simulink model "TorqueVectoring_6_1"  (R2023a)
settings: Solver=FixedStepAuto  StartTime=0.0  StopTime=8  FixedStep=.001  RelTol=1e-3
model workspace (MAT data in the model file):
  slipTarget : Simulink.Parameter (value not decoded)
values from neighbouring files (symbols this model uses):
  Kd_slip = 0    [Main_TorqueVectoring_5_1.m]
  Kd_yaw = 0    [Main_TorqueVectoring_5_1.m]
  Ki_slip = 50    [Main_TorqueVectoring_5_1.m]
  Ki_yaw = 10    [Main_TorqueVectoring_5_1.m]
  Kp_slip = 250    [Main_TorqueVectoring_5_1.m]
  Kp_yaw = 100    [Main_TorqueVectoring_5_1.m]
  slip_windupLower = -inf    [Main_TorqueVectoring_5_1.m]
  slip_windupUpper = inf    [Main_TorqueVectoring_5_1.m]
  slipTarget = .2    (= 0.2)    [Main_TorqueVectoring_5_1.m]
  steering = table2array(yawrateSteering)    [Main_TorqueVectoring_5_1.m]
  yaw_prev_error = 0    [Main_TorqueVectoring_5_1.m]
  yawRate = table2array(yawrateTable)    [Main_TorqueVectoring_5_1.m]
  yawrateVelocity = [0, 5, 10, 15, 20, 25, 30, 35]    [Main_TorqueVectoring_5_1.m]
undefined symbols (not defined in the file or in its folder): sigbuilder_block, VehicleVelocity
libraries: slpidlib x6
(part 2 of 4)

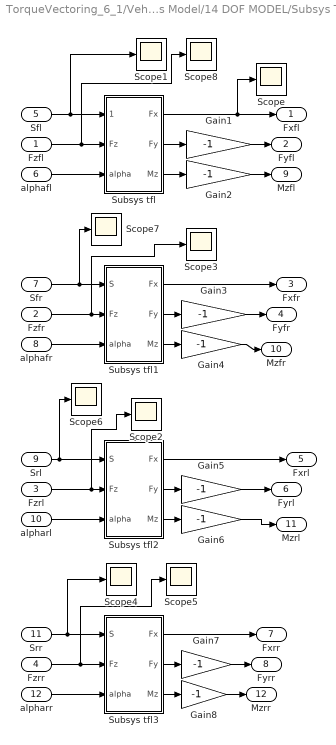
== system TorqueVectoring_6_1/Vehicle Dynamics Model/14 DOF MODEL/Subsys Tire ==
  Fzfl : Inport
  Fzfr : Inport  Port=2
  Fzrl : Inport  Port=3
  Fzrr : Inport  Port=4
  Sfl : Inport  Port=5
  alphafl : Inport  Port=6
  Sfr : Inport  Port=7
  alphafr : Inport  Port=8
  Srl : Inport  Port=9
  alpharl : Inport  Port=10
  Srr : Inport  Port=11
  alpharr : Inport  Port=12
  Gain{1..8} (8 alike) : Gain  Gain=-1
  Scope{,1..8} (9 alike) : Scope
  Subsys tfl : Subsystem
  Subsys tfl1 : Subsystem
  Subsys tfl2 : Subsystem
  Subsys tfl3 : Subsystem
  Fxfl : Outport
  Fyfl : Outport  Port=2
  Fxfr : Outport  Port=3
  Fyfr : Outport  Port=4
  Fxrl : Outport  Port=5
  Fyrl : Outport  Port=6
  Fxrr : Outport  Port=7
  Fyrr : Outport  Port=8
  Mzfl : Outport  Port=9
  Mzfr : Outport  Port=10
  Mzrl : Outport  Port=11
  Mzrr : Outport  Port=12
  wires:
  Subsys tfl/1(Fx) -> Scope/1, Fxfl/1
  Subsys tfl/2(Fy) -> Gain1/1
  Subsys tfl/3(Mz) -> Gain2/1
  Sfl/1 -> Scope1/1, Subsys tfl/1(Slip Ratio)
  Fzfl/1 -> Scope8/1, Subsys tfl/2(Fz)
  alphafl/1 -> Subsys tfl/3(alpha)
  Subsys tfl1/1(Fx) -> Fxfr/1
  Subsys tfl1/2(Fy) -> Gain3/1
  Subsys tfl1/3(Mz) -> Gain4/1
  alphafr/1 -> Subsys tfl1/3(alpha)
  Subsys tfl2/1(Fx) -> Fxrl/1
  Subsys tfl2/2(Fy) -> Gain5/1
  Subsys tfl2/3(Mz) -> Gain6/1
  Srl/1 -> Subsys tfl2/1(S), Scope6/1
  Fzrl/1 -> Scope2/1, Subsys tfl2/2(Fz)
  alpharl/1 -> Subsys tfl2/3(alpha)
  Subsys tfl3/1(Fx) -> Fxrr/1
  Subsys tfl3/2(Fy) -> Gain7/1
  Subsys tfl3/3(Mz) -> Gain8/1
  Srr/1 -> Scope4/1, Subsys tfl3/1(S)
  Fzrr/1 -> Scope5/1, Subsys tfl3/2(Fz)
  alpharr/1 -> Subsys tfl3/3(alpha)
  Gain1/1 -> Fyfl/1
  Gain2/1 -> Mzfl/1
  Gain3/1 -> Fyfr/1
  Gain4/1 -> Mzfr/1
  Gain5/1 -> Fyrl/1
  Gain6/1 -> Mzrl/1
  Gain7/1 -> Fyrr/1
  Gain8/1 -> Mzrr/1
  Fzfr/1 -> Subsys tfl1/2(Fz), Scope3/1
  Sfr/1 -> Scope7/1, Subsys tfl1/1(S)

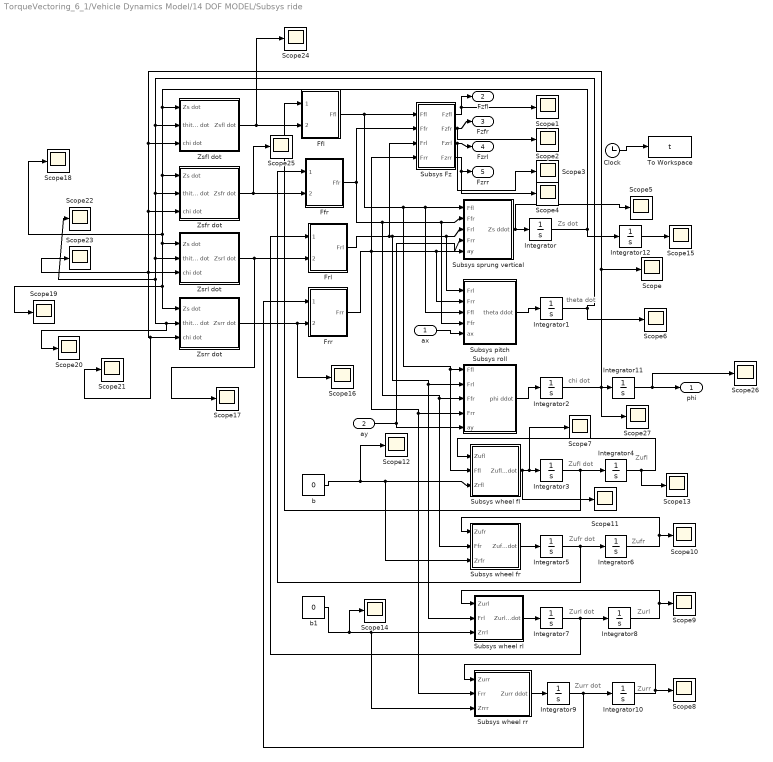
== system TorqueVectoring_6_1/Vehicle Dynamics Model/14 DOF MODEL/Subsys ride ==
  note: Zs dot
  note: theta dot
  note: chi dot
  note: Zufl dot
  note: Zufr dot
  note: Zurl dot
  note: Zurr dot
  note: Zufl
  note: Zufr
  note: Zurl
  note: Zurr
  ax : Inport
  ay : Inport  Port=2
  Clock : Clock
  Ffl : Subsystem
  Ffr : Subsystem
  Frl : Subsystem
  Frr : Subsystem
  Integrator{,1..12} (13 alike) : Integrator
  Scope{,1..27} (28 alike) : Scope
  Subsys Fz : Subsystem
  Subsys pitch : Subsystem
  Subsys roll : Subsystem
  Subsys sprung vertical : Subsystem
  Subsys wheel fl : Subsystem
  Subsys wheel fr : Subsystem
  Subsys wheel rl : Subsystem
  Subsys wheel rr : Subsystem
  To Workspace : ToWorkspace  VariableName=t  SampleTime=-1
  Zsfl dot : Subsystem
  Zsfr dot : Subsystem
  Zsrl dot : Subsystem
  Zsrr dot : Subsystem
  b : Constant  Value=0
  b1 : Constant  Value=0
  phi : Outport
  Fzfl : Outport  Port=2
  Fzfr : Outport  Port=3
  Fzrl : Outport  Port=4
  Fzrr : Outport  Port=5
  wires:
  Ffl/1(Ffl) -> Subsys sprung vertical/1(Ffl), Subsys pitch/3(Ffl), Subsys wheel fl/2(Ffl), Subsys roll/1(Ffl), Subsys Fz/1(Ffl)
  Ffr/1(Ffr) -> Subsys sprung vertical/2(Ffr), Subsys pitch/4(Ffr), Subsys wheel fr/2(Ffr), Subsys roll/3(Ffr), Subsys Fz/2(Ffr)
  Frl/1(Frl) -> Subsys sprung vertical/3(Frl), Subsys pitch/1(Frl), Subsys wheel rl/2(Frl), Subsys roll/2(Frl), Subsys Fz/3(Frl)
  Frr/1(Frr) -> Subsys sprung vertical/4(Frr), Subsys pitch/2(Frr), Subsys wheel rr/2(Frr), Subsys roll/4(Frr), Subsys Fz/4(Frr)
  Subsys sprung vertical/1(Zs ddot) -> Integrator/1, Scope5/1
  Integrator/1 -> Zsrl dot/1(Zs dot), Zsrr dot/1(Zs dot), Scope19/1, Scope18/1, Zsfr dot/1(Zs dot), Zsfl dot/1(Zs dot), Integrator12/1
  Zsfr dot/1(Zsfr dot) -> Scope25/1, Ffr/2(Zsfr dot)
  Zsfl dot/1(Zsfl dot) -> Scope24/1, Ffl/2(Zsfl dot)
  Zsrl dot/1(Zsrl dot) -> Frl/2(Zsrl dot), Scope17/1
  Zsrr dot/1(Zsrr dot) -> Scope16/1, Frr/2(Zsrr dot)
  Subsys pitch/1(theta ddot) -> Integrator1/1
  Subsys roll/1(phi ddot) -> Integrator2/1
  Integrator2/1 -> Scope27/1, Zsrl dot/3(chi dot), Scope23/1, Scope21/1, Zsrr dot/3(chi dot), Zsfr dot/3(chi dot), Zsfl dot/3(chi dot), Scope/1, Integrator11/1
  Subsys wheel fl/1(Zufl ddot) -> Integrator3/1, Scope7/1, Scope11/1
  Integrator3/1 -> Integrator4/1, Ffl/1(Zufl dot)
  Subsys wheel fr/1(Zufr ddot) -> Integrator5/1
  Integrator5/1 -> Integrator6/1, Ffr/1(Zufr dot)
  Subsys wheel rl/1(Zurl ddot) -> Integrator7/1
  Integrator7/1 -> Integrator8/1, Frl/1(Zurl dot)
  Subsys wheel rr/1(Zurr ddot) -> Integrator9/1
  Integrator9/1 -> Integrator10/1, Frr/1(Zurr dot)
  Integrator4/1 -> Subsys wheel fl/1(Zufl), Scope13/1
  Integrator6/1 -> Subsys wheel fr/1(Zufr), Scope10/1
  Integrator8/1 -> Scope9/1, Subsys wheel rl/1(Zurl)
  Integrator10/1 -> Scope8/1, Subsys wheel rr/1(Zurr)
  Clock/1 -> To Workspace/1
  Integrator1/1 -> Scope22/1, Scope20/1, Zsrr dot/2(thita dot), Zsrl dot/2(thita dot), Zsfr dot/2(thita dot), Zsfl dot/2(thita dot), Scope6/1
  Subsys Fz/1(Fzfl) -> Fzfl/1, Scope1/1
  Subsys Fz/2(Fzfr) -> Fzfr/1, Scope2/1
  Subsys Fz/3(Fzrl) -> Fzrl/1, Scope3/1
  Subsys Fz/4(Fzrr) -> Fzrr/1, Scope4/1
  b/1 -> Subsys wheel fl/3(Zrfl), Subsys wheel fr/3(Zrfr), Scope12/1
  b1/1 -> Subsys wheel rl/3(Zrrl), Subsys wheel rr/3(Zrrr), Scope14/1
  ay/1 -> Subsys roll/5(ay), Subsys sprung vertical/5(ay)
  ax/1 -> Subsys pitch/5(ax)
  Integrator11/1 -> Scope26/1, phi/1
  Integrator12/1 -> Scope15/1

== system TorqueVectoring_6_1/Vehicle Dynamics Model/14 DOF MODEL/degree conversion ==
  alpha(degree) : Inport
  180 degrees : Constant  Value=180
  Divide : Product  Inputs=**/
  pi : Constant  Value=22/7
  alpha(rad) : Outport
  wires:
  alpha(degree)/1 -> Divide/1
  Divide/1 -> alpha(rad)/1
  pi/1 -> Divide/2
  180 degrees/1 -> Divide/3

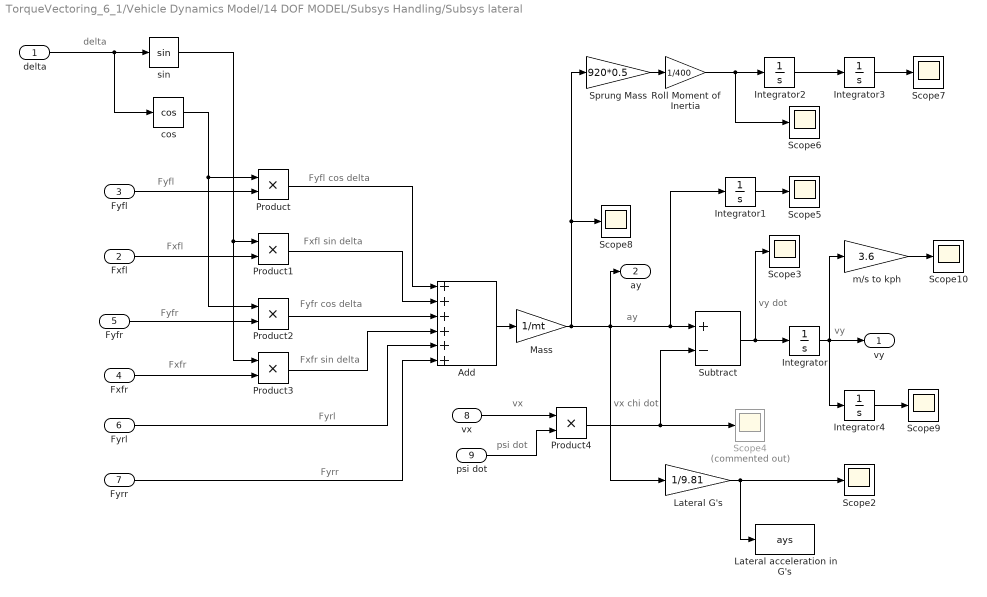
== system TorqueVectoring_6_1/Vehicle Dynamics Model/14 DOF MODEL/Subsys Handling/Subsys lateral ==
  note: vy
  note: vy dot
  note: ay
  note: vx
  note: delta
  note: Fyrr
  note: Fyrl
  note: Fxfr
  note: Fyfr
  note: Fxfl
  note: Fyfl
  note: Fyfl cos delta
  note: Fxfl sin delta
  note: Fyfr cos delta
  note: Fxfr sin delta
  note: vx chi dot
  note: psi dot
  delta : Inport
  Fxfl : Inport  Port=2
  Fyfl : Inport  Port=3
  Fxfr : Inport  Port=4
  Fyfr : Inport  Port=5
  Fyrl : Inport  Port=6
  Fyrr : Inport  Port=7
  vx : Inport  Port=8
  "psi dot " : Inport  Port=9
  Add : Sum  Inputs=++++++
  Integrator{,1..4} (5 alike) : Integrator
  Lateral G's : Gain  Gain=1/9.81
  Lateral acceleration in G's : ToWorkspace  VariableName=ays  SampleTime=-1
  Mass : Gain  Gain=1/mt
  Product{,1..4} (5 alike) : Product  RndMeth=Zero
  Roll Moment of Inertia : Gain  Gain=1/400
  Scope{2..3,5..10} (8 alike) : Scope
  Scope4 : Scope  Commented=on
  Sprung Mass : Gain  Gain=920*0.5
  Subtract : Sum  Inputs=+-
  cos : Trigonometry  Operator=cos
  m/s to kph : Gain  Gain=3.6
  sin : Trigonometry
  vy : Outport
  ay : Outport  Port=2
  wires:
  Integrator/1 -> vy/1, Integrator4/1, m/s to kph/1
  Subtract/1 -> Integrator/1, Scope3/1
  Product4/1 -> Subtract/2, Scope4/1
  Mass/1 -> Subtract/1, Integrator1/1, ay/1, Lateral G's/1, Sprung Mass/1, Scope8/1
  vx/1 -> Product4/1
  Add/1 -> Mass/1
  Fyrr/1 -> Add/6
  Fyrl/1 -> Add/5
  Product3/1 -> Add/4
  Product2/1 -> Add/3
  Product1/1 -> Add/2
  Product/1 -> Add/1
  Fxfr/1 -> Product3/2
  Fyfr/1 -> Product2/2
  Fxfl/1 -> Product1/2
  Fyfl/1 -> Product/2
  sin/1 -> Product1/1, Product3/1
  cos/1 -> Product2/1, Product/1
  delta/1 -> cos/1, sin/1
  Integrator1/1 -> Scope5/1
  "psi dot "/1 -> Product4/2
  Lateral G's/1 -> Scope2/1, Lateral acceleration in G's/1
  Sprung Mass/1 -> Roll Moment of Inertia/1
  Integrator2/1 -> Integrator3/1
  Integrator3/1 -> Scope7/1
  Roll Moment of Inertia/1 -> Scope6/1, Integrator2/1
  Integrator4/1 -> Scope9/1
  m/s to kph/1 -> Scope10/1

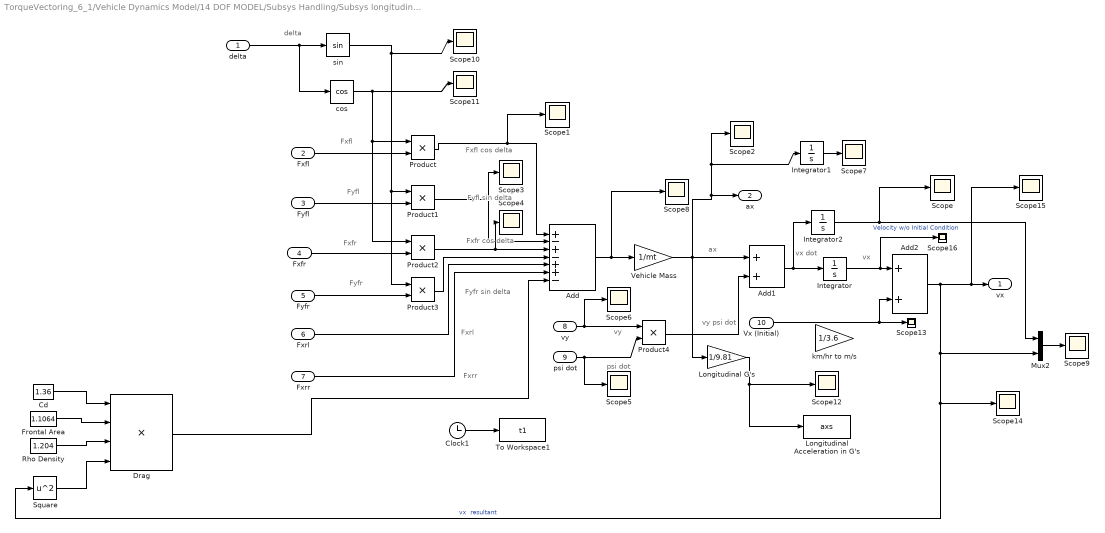
== system TorqueVectoring_6_1/Vehicle Dynamics Model/14 DOF MODEL/Subsys Handling/Subsys longitudinal ==
  note: Fxfl
  note: Fyfl
  note: Fxfr
  note: Fyfr
  note: Fxrl
  note: Fxrr
  note: delta
  note: vy
  note: ax
  note: vx dot
  note: vx
  note: Fxfl cos delta
  note: Fyfl sin delta
  note: Fxfr cos delta
  note: Fyfr sin delta
  note: psi dot
  note: vy psi dot
  delta : Inport
  Fxfl : Inport  Port=2
  Fyfl : Inport  Port=3
  Fxfr : Inport  Port=4
  Fyfr : Inport  Port=5
  Fxrl : Inport  Port=6
  Fxrr : Inport  Port=7
  vy : Inport  Port=8
  "psi dot " : Inport  Port=9
  Vx (Initial) : Inport  Port=10
  Add : Sum  Inputs=+-+-++-
  Add1 : Sum
  Add2 : Sum
  Cd : Constant  Value=1.36
  Clock1 : Clock
  Drag : Product  Inputs=4
  Frontal Area : Constant  Value=1.1064
  Integrator : Integrator
  Integrator1 : Integrator
  Integrator2 : Integrator  InitialCondition=50/3.6
  Longitudinal Acceleration in G's : ToWorkspace  VariableName=axs  SampleTime=-1
  Longitudinal G's : Gain  Gain=1/9.81
  Mux2 : Mux  Inputs=2
  Product{,1..4} (5 alike) : Product  RndMeth=Zero
  Rho Density : Constant  Value=1.204
  Scope{,1..16} (17 alike) : Scope
  Square : Math  Operator=square
  To Workspace1 : ToWorkspace  VariableName=t1  SampleTime=-1
  Vehicle Mass : Gain  Gain=1/mt
  cos : Trigonometry  Operator=cos
  km/hr to m/s : Gain  Gain=1/3.6
  sin : Trigonometry
  vx : Outport
  ax : Outport  Port=2
  wires:
  delta/1 -> sin/1, cos/1
  cos/1 -> Product/1, Product2/1, Scope11/1
  sin/1 -> Product3/1, Product1/1, Scope10/1
  Fxfl/1 -> Product/2
  Fyfl/1 -> Product1/2
  Fxfr/1 -> Product2/2
  Fyfr/1 -> Product3/2
  Product/1 -> Add/1, Scope1/1
  Product1/1 -> Add/2, Scope3/1
  Product2/1 -> Add/3, Scope4/1
  Product3/1 -> Add/4
  Fxrl/1 -> Add/5
  Fxrr/1 -> Add/6
  Add/1 -> Vehicle Mass/1, Scope8/1
  "psi dot "/1 -> Product4/2, Scope5/1
  vy/1 -> Product4/1, Scope6/1
  Vehicle Mass/1 -> ax/1, Scope2/1, Integrator1/1, Longitudinal G's/1, Add1/1
  Add1/1 -> Integrator/1, Integrator2/1
  Integrator/1 -> Scope16/1, Add2/1
  Product4/1 -> Add1/2
  Integrator1/1 -> Scope7/1
  Longitudinal G's/1 -> Longitudinal Acceleration in G's/1, Scope12/1
  Clock1/1 -> To Workspace1/1
  Add2/1 -> Scope15/1, vx/1, Square/1, Scope14/1, Mux2/2  "vx  resultant"
  Mux2/1 -> Scope9/1
  Integrator2/1 -> Mux2/1, Scope/1  "Velocity w/o Initial Condition"
  Vx (Initial)/1 -> Scope13/1, Add2/2
  Drag/1 -> Add/7
  Frontal Area/1 -> Drag/2
  Cd/1 -> Drag/1
  Rho Density/1 -> Drag/3
  Square/1 -> Drag/4

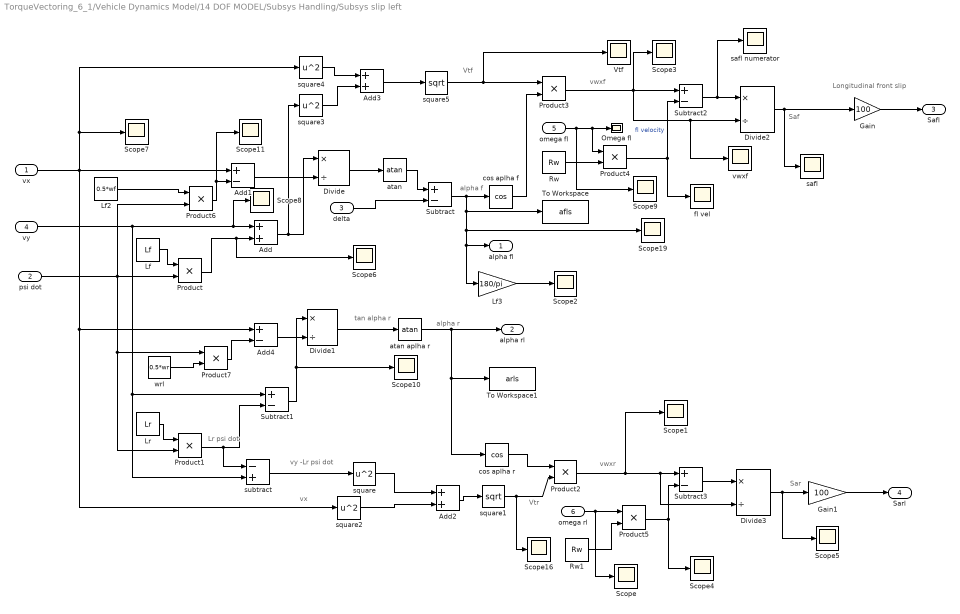
== system TorqueVectoring_6_1/Vehicle Dynamics Model/14 DOF MODEL/Subsys Handling/Subsys slip left  ==
  note: tan alpha r
  note: alpha r
  note: Lr psi dot
  note: vx
  note: vy -Lr psi dot
  note: Vtr
  note: alpha f
  note: vwxr
  note: Vtf
  note: vwxf
  note: Saf
  note: Longitudinal front slip
  note: Sar
  vx : Inport
  psi dot : Inport  Port=2
  delta : Inport  Port=3
  vy : Inport  Port=4
  omega fl : Inport  Port=5
  omega rl : Inport  Port=6
  Add : Sum
  Add1 : Sum  Inputs=+-
  Add2 : Sum
  Add3 : Sum
  Add4 : Sum  Inputs=+-
  Divide{,1..3} (4 alike) : Product  Inputs=*/
  Gain : Gain  Gain=100
  Gain1 : Gain  Gain=100
  Lf : Constant  Value=Lf
  Lf2 : Constant  Value=0.5*wf
  Lf3 : Gain  Gain=180/pi
  Lr : Constant  Value=Lr
  Omega fl : Scope
  Product{,1..7} (8 alike) : Product  RndMeth=Zero
  Rw : Constant  Value=Rw
  Rw1 : Constant  Value=Rw
  Scope{,1..11,16,19} (14 alike) : Scope
  Subtract{,1..3} (4 alike) : Sum  Inputs=+-
  To Workspace : ToWorkspace  VariableName=afls  SampleTime=-1
  To Workspace1 : ToWorkspace  VariableName=arls  SampleTime=-1
  Vtf : Scope
  "atan " : Trigonometry  Operator=atan
  atan aplha r : Trigonometry  Operator=atan
  cos aplha f : Trigonometry  Operator=cos
  cos aplha r : Trigonometry  Operator=cos
  fl vel : Scope
  safl : Scope
  safl numerator : Scope
  square{,2..4} (4 alike) : Math  Operator=square  SignedPower=on
  square1 : Math  Operator=sqrt  SignedPower=on
  square5 : Math  Operator=sqrt  SignedPower=on
  subtract : Sum  Inputs=-+
  vwxf : Scope
  wrl : Constant  Value=0.5*wr
  alpha fl : Outport
  alpha rl : Outport  Port=2
  Safl : Outport  Port=3
  Sarl : Outport  Port=4
  wires:
  Lf/1 -> Product/1
  psi dot/1 -> Product/2, Product6/2, Product1/2, Product7/1
  Add/1 -> Divide/1, square3/1
  delta/1 -> Subtract/2
  vx/1 -> Scope7/1, square4/1, Add1/1, square2/1, Add4/1
  Product/1 -> Scope6/1, Add/2
  vy/1 -> Subtract1/1, subtract/2, Scope8/1, Add/1
  Divide/1 -> "atan "/1
  "atan "/1 -> Subtract/1
  Subtract1/1 -> Divide1/1, Scope10/1
  Lr/1 -> Product1/1
  Product1/1 -> subtract/1, Subtract1/2
  Divide1/1 -> atan aplha r/1
  atan aplha r/1 -> To Workspace1/1, cos aplha r/1, alpha rl/1
  subtract/1 -> square/1
  square/1 -> Add2/1
  square2/1 -> Add2/2
  Add2/1 -> square1/1
  square1/1 -> Product2/2, Scope16/1
  cos aplha r/1 -> Product2/1
  Product2/1 -> Scope1/1, Subtract3/1, Divide3/2
  square4/1 -> Add3/1
  square3/1 -> Add3/2
  Add3/1 -> square5/1
  Subtract/1 -> Lf3/1, alpha fl/1, Scope19/1, To Workspace/1, cos aplha f/1
  square5/1 -> Vtf/1, Product3/1
  cos aplha f/1 -> Product3/2
  Product3/1 -> vwxf/1, Divide2/2, Subtract2/1, Scope3/1
  omega fl/1 -> Scope9/1, Omega fl/1, Product4/1
  Rw/1 -> Product4/2
  Product4/1 -> Subtract2/2, fl vel/1  "fl velocity"
  Subtract2/1 -> safl numerator/1, Divide2/1
  omega rl/1 -> Scope/1, Product5/1
  Rw1/1 -> Product5/2
  Product5/1 -> Subtract3/2, Scope4/1
  Subtract3/1 -> Divide3/1
  Divide3/1 -> Scope5/1, Gain1/1
  Divide2/1 -> Gain/1, safl/1
  Add1/1 -> Divide/2
  Product6/1 -> Scope11/1, Add1/2
  Lf2/1 -> Product6/1
  wrl/1 -> Product7/2
  Add4/1 -> Divide1/2
  Product7/1 -> Add4/2
  Lf3/1 -> Scope2/1
  Gain/1 -> Safl/1
  Gain1/1 -> Sarl/1

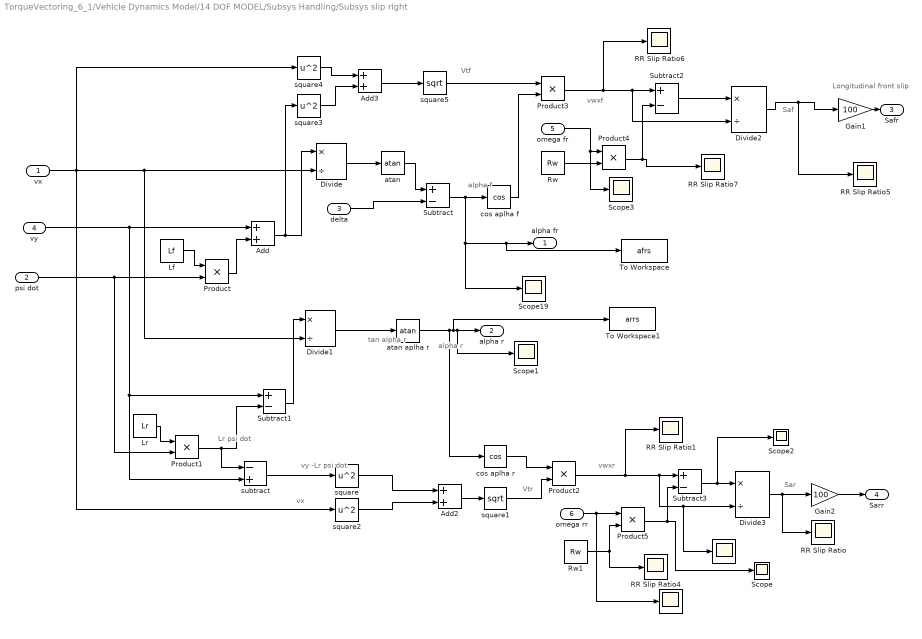
== system TorqueVectoring_6_1/Vehicle Dynamics Model/14 DOF MODEL/Subsys Handling/Subsys slip right ==
  note: Sar
  note: Longitudinal front slip
  note: Saf
  note: vwxf
  note: Vtf
  note: vwxr
  note: alpha f
  note: Vtr
  note: vy -Lr psi dot
  note: vx
  note: Lr psi dot
  note: alpha r
  note: tan alpha r
  vx : Inport
  psi dot : Inport  Port=2
  delta : Inport  Port=3
  vy : Inport  Port=4
  omega fr : Inport  Port=5
  omega rr : Inport  Port=6
  " " : Scope
  "  " : Scope
  Add : Sum
  Add2 : Sum
  Add3 : Sum
  Divide{,1..3} (4 alike) : Product  Inputs=*/
  Gain1 : Gain  Gain=100
  Gain2 : Gain  Gain=100
  Lf : Constant  Value=Lf
  Lr : Constant  Value=Lr
  Product{,1..5} (6 alike) : Product  RndMeth=Zero
  RR Slip Ratio{,1,4..7} (6 alike) : Scope
  Rw : Constant  Value=Rw
  Rw1 : Constant  Value=Rw
  Scope{,1..3,19} (5 alike) : Scope
  Subtract{,1..3} (4 alike) : Sum  Inputs=+-
  To Workspace : ToWorkspace  VariableName=afrs  SampleTime=-1
  To Workspace1 : ToWorkspace  VariableName=arrs  SampleTime=-1
  "atan " : Trigonometry  Operator=atan
  atan aplha r : Trigonometry  Operator=atan
  cos aplha f : Trigonometry  Operator=cos
  cos aplha r : Trigonometry  Operator=cos
  square{,2..4} (4 alike) : Math  Operator=square  SignedPower=on
  square1 : Math  Operator=sqrt  SignedPower=on
  square5 : Math  Operator=sqrt  SignedPower=on
  subtract : Sum  Inputs=-+
  alpha fr : Outport
  alpha r : Outport  Port=2
  Safr : Outport  Port=3
  Sarr : Outport  Port=4
  wires:
  Divide3/1 -> RR Slip Ratio/1, Gain2/1
  Subtract3/1 -> Scope2/1, Divide3/1
  Product5/1 -> Subtract3/2, Scope/1
  Rw1/1 -> Product5/2, RR Slip Ratio4/1
  omega rr/1 -> "  "/1, Product5/1
  Divide2/1 -> RR Slip Ratio5/1, Gain1/1
  Subtract2/1 -> Divide2/1
  Product4/1 -> RR Slip Ratio7/1, Subtract2/2
  Rw/1 -> Product4/2
  omega fr/1 -> Scope3/1, Product4/1
  Product3/1 -> RR Slip Ratio6/1, Divide2/2, Subtract2/1
  cos aplha f/1 -> Product3/2
  square5/1 -> Product3/1
  Subtract/1 -> cos aplha f/1, Scope19/1, alpha fr/1, To Workspace/1
  Add3/1 -> square5/1
  square3/1 -> Add3/2
  square4/1 -> Add3/1
  Product2/1 -> RR Slip Ratio1/1, Subtract3/1, " "/1, Divide3/2
  cos aplha r/1 -> Product2/1
  square1/1 -> Product2/2
  Add2/1 -> square1/1
  square2/1 -> Add2/2
  square/1 -> Add2/1
  subtract/1 -> square/1
  atan aplha r/1 -> cos aplha r/1, alpha r/1, Scope1/1, To Workspace1/1
  Divide1/1 -> atan aplha r/1
  Product1/1 -> subtract/1, Subtract1/2
  Lr/1 -> Product1/1
  Subtract1/1 -> Divide1/1
  "atan "/1 -> Subtract/1
  Divide/1 -> "atan "/1
  vy/1 -> subtract/2, Subtract1/1, Add/1
  Product/1 -> Add/2
  vx/1 -> square4/1, Divide1/2, Divide/2, square2/1
  delta/1 -> Subtract/2
  Add/1 -> square3/1, Divide/1
  psi dot/1 -> Product1/2, Product/2
  Lf/1 -> Product/1
  Gain1/1 -> Safr/1
  Gain2/1 -> Sarr/1

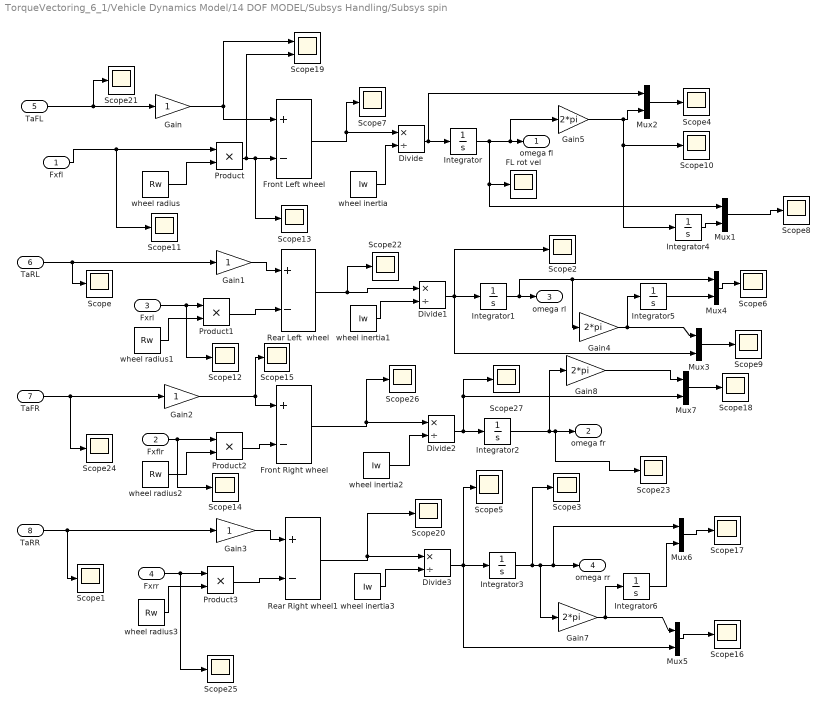
== system TorqueVectoring_6_1/Vehicle Dynamics Model/14 DOF MODEL/Subsys Handling/Subsys spin ==
  Fxfl : Inport
  Fxflr : Inport  Port=2
  Fxrl : Inport  Port=3
  Fxrr : Inport  Port=4
  TaFL : Inport  Port=5
  TaRL : Inport  Port=6
  TaFR : Inport  Port=7
  TaRR : Inport  Port=8
  Divide{,1..3} (4 alike) : Product  Inputs=*/
  FL rot vel : Scope
  Front Left wheel : Sum  Inputs=+-
  Front Right wheel : Sum  Inputs=+-
  Gain{,1..3} (4 alike) : Gain
  Gain{4..5,7..8} (4 alike) : Gain  Gain=2*pi
  Integrator{,1..6} (7 alike) : Integrator
  Mux{1..7} (7 alike) : Mux  Inputs=2
  Product{,1..3} (4 alike) : Product  RndMeth=Zero
  Rear Left  wheel : Sum  Inputs=+-
  Rear Right wheel1 : Sum  Inputs=+-
  Scope{,1..18,20..27} (27 alike) : Scope
  Scope19 : Scope  NumInputPorts=2
  wheel inertia{,1..3} (4 alike) : Constant  Value=Iw
  wheel radius{,1..3} (4 alike) : Constant  Value=Rw
  omega fl : Outport
  omega fr : Outport  Port=2
  omega rl : Outport  Port=3
  omega rr : Outport  Port=4
  wires:
  TaFL/1 -> Scope21/1, Gain/1
  Gain1/1 -> Rear Left  wheel/1
  Gain/1 -> Scope19/1, Front Left wheel/1
  Front Left wheel/1 -> Divide/1, Scope7/1
  Rear Left  wheel/1 -> Scope22/1, Divide1/1
  Product1/1 -> Rear Left  wheel/2
  wheel inertia/1 -> Divide/2
  wheel inertia1/1 -> Divide1/2
  Divide/1 -> Integrator/1, Mux2/1
  Divide1/1 -> Integrator1/1, Scope2/1, Mux3/2
  Fxfl/1 -> Product/1, Scope11/1
  Product/1 -> Scope19/2, Front Left wheel/2, Scope13/1
  wheel radius/1 -> Product/2
  Fxrl/1 -> Product1/1, Scope12/1
  wheel radius1/1 -> Product1/2
  Gain2/1 -> Front Right wheel/1, Scope15/1
  wheel inertia2/1 -> Divide2/2
  Fxflr/1 -> Product2/1, Scope14/1
  Product2/1 -> Front Right wheel/2
  wheel radius2/1 -> Product2/2
  Gain3/1 -> Rear Right wheel1/1
  Rear Right wheel1/1 -> Divide3/1, Scope20/1
  Product3/1 -> Rear Right wheel1/2
  wheel inertia3/1 -> Divide3/2
  Divide3/1 -> Integrator3/1, Scope5/1, Mux5/2
  Fxrr/1 -> Scope25/1, Product3/1
  wheel radius3/1 -> Product3/2
  Mux1/1 -> Scope8/1
  Integrator/1 -> Mux1/1, FL rot vel/1, Gain5/1, omega fl/1
  Gain5/1 -> Integrator4/1, Scope10/1, Mux2/2
  Mux2/1 -> Scope4/1
  Integrator4/1 -> Mux1/2
  Mux3/1 -> Scope9/1
  Integrator1/1 -> omega rl/1, Gain4/1, Mux4/1
  Gain4/1 -> Mux3/1, Integrator5/1
  Integrator5/1 -> Mux4/2
  Mux4/1 -> Scope6/1
  Mux5/1 -> Scope16/1
  Integrator3/1 -> Scope3/1, Gain7/1, omega rr/1, Mux6/1
  Gain7/1 -> Mux5/1, Integrator6/1
  Integrator6/1 -> Mux6/2
  Mux6/1 -> Scope17/1
  Mux7/1 -> Scope18/1
  Gain8/1 -> Mux7/1
  Integrator2/1 -> Gain8/1, Scope23/1, omega fr/1
  TaRR/1 -> Scope1/1, Gain3/1
  TaFR/1 -> Scope24/1, Gain2/1
  TaRL/1 -> Scope/1, Gain1/1
  Front Right wheel/1 -> Scope26/1, Divide2/1
  Divide2/1 -> Integrator2/1, Scope27/1, Mux7/2

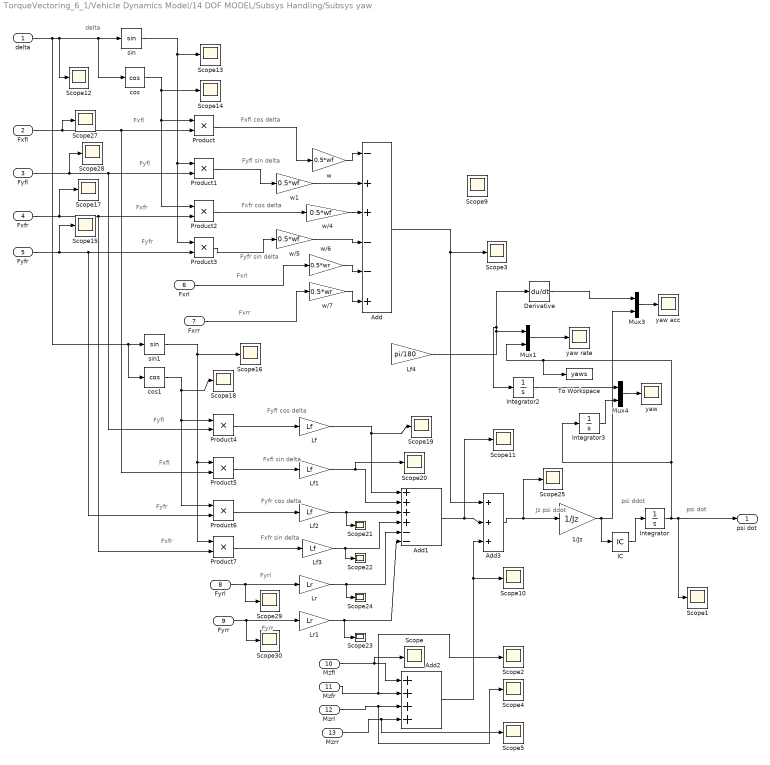
== system TorqueVectoring_6_1/Vehicle Dynamics Model/14 DOF MODEL/Subsys Handling/Subsys yaw  ==
  note: Fxfl
  note: Fyfl
  note: Fxfr
  note: Fyfr
  note: Fxrl
  note: Fxrr
  note: delta
  note: Fxfl cos delta
  note: Fyfl sin delta
  note: Fxfr cos delta
  note: Fyfr sin delta
  note: Fyrr
  note: Fyrl
  note: Fxfr
  note: Fyfr
  note: Fxfl
  note: Fyfl
  note: Fyfl cos delta
  note: Fxfl sin delta
  note: Fyfr cos delta
  note: Fxfr sin delta
  note: Jz psi ddot
  note: psi ddot
  note: psi dot
  delta : Inport
  Fxfl : Inport  Port=2
  Fyfl : Inport  Port=3
  Fxfr : Inport  Port=4
  Fyfr : Inport  Port=5
  Fxrl : Inport  Port=6
  Fxrr : Inport  Port=7
  Fyrl : Inport  Port=8
  Fyrr : Inport  Port=9
  Mzfl : Inport  Port=10
  Mzfr : Inport  Port=11
  Mzrl : Inport  Port=12
  Mzrr : Inport  Port=13
  1/Jz : Gain  Gain=1/Jz
  Add : Sum  Inputs=-++--+
  Add1 : Sum  Inputs=++++--
  Add2 : Sum  Inputs=++++
  Add3 : Sum  Inputs=+++
  Derivative : Derivative
  IC : InitialCondition  Value=0
  Integrator : Integrator
  Integrator2 : Integrator
  Integrator3 : Integrator
  Lf{,1..3} (4 alike) : Gain  Gain=Lf
  Lf4 : Gain  Gain=pi/180
  Lr : Gain  Gain=Lr
  Lr1 : Gain  Gain=Lr
  Mux1 : Mux  Inputs=2
  Mux3 : Mux  Inputs=2
  Mux4 : Mux  Inputs=2
  Product{,1..7} (8 alike) : Product  RndMeth=Zero
  Scope{,1..5,9..25,27..30} (27 alike) : Scope
  To Workspace : ToWorkspace  VariableName=yaws  SampleTime=-1
  cos : Trigonometry  Operator=cos
  cos1 : Trigonometry  Operator=cos
  sin : Trigonometry
  sin1 : Trigonometry
  w : Gain  Gain=0.5*wf
  w/4 : Gain  Gain=0.5*wf
  w/5 : Gain  Gain=0.5*wf
  w/6 : Gain  Gain=0.5*wr
  w/7 : Gain  Gain=0.5*wr
  w1 : Gain  Gain=0.5*wf
  yaw : Scope
  yaw acc : Scope
  yaw rate : Scope
  psi dot : Outport
  wires:
  delta/1 -> sin1/1, cos1/1, sin/1, cos/1, Scope12/1
  cos/1 -> Product/1, Product2/1, Scope14/1
  sin/1 -> Product3/1, Product1/1, Scope13/1
  Fxfl/1 -> Product/2, Product5/2, Scope27/1
  Fyfl/1 -> Product1/2, Product4/2, Scope28/1
  Fxfr/1 -> Product2/2, Product7/2, Scope17/1
  Fyfr/1 -> Product3/2, Product6/2, Scope15/1
  Product2/1 -> w/4/1
  Product3/1 -> w/5/1
  Fxrl/1 -> w/6/1
  Fxrr/1 -> w/7/1
  Product1/1 -> w1/1
  Product/1 -> w/1
  sin1/1 -> Product5/1, Product7/1, Scope16/1
  cos1/1 -> Product6/1, Product4/1, Scope18/1
  Product4/1 -> Lf/1
  Lf/1 -> Add1/1, Scope19/1
  Product5/1 -> Lf1/1
  Product6/1 -> Lf2/1
  Product7/1 -> Lf3/1
  Lf1/1 -> Add1/2, Scope20/1
  Lf2/1 -> Add1/3, Scope21/1
  Lf3/1 -> Add1/4, Scope22/1
  Fyrr/1 -> Lr1/1, Scope30/1
  Lr/1 -> Add1/5, Scope24/1
  Lr1/1 -> Add1/6, Scope23/1
  Add/1 -> Add3/1, Scope3/1
  Fyrl/1 -> Lr/1, Scope29/1
  Integrator/1 -> Integrator3/1, Mux1/2, To Workspace/1, Scope1/1, psi dot/1
  1/Jz/1 -> IC/1, Mux3/2
  Add3/1 -> 1/Jz/1, Scope25/1
  Add1/1 -> Scope11/1, Add3/2
  ? -> Lf4/1
  Mux1/1 -> yaw rate/1
  w/1 -> Add/1
  w1/1 -> Add/2
  w/4/1 -> Add/3
  w/5/1 -> Add/4
  w/6/1 -> Add/5
  w/7/1 -> Add/6
  Mzfl/1 -> Scope/1, Add2/1
  Mzfr/1 -> Scope2/1, Add2/2
  Add2/1 -> Scope10/1, Add3/3
  Mzrl/1 -> Scope4/1, Add2/3
  Mzrr/1 -> Scope5/1, Add2/4
  Lf4/1 -> Derivative/1, Integrator2/1, Mux1/1
  Mux3/1 -> yaw acc/1
  Derivative/1 -> Mux3/1
  Integrator2/1 -> Mux4/1
  Integrator3/1 -> Mux4/2
  Mux4/1 -> yaw/1
  IC/1 -> Integrator/1

== system TorqueVectoring_6_1/Vehicle Dynamics Model/14 DOF MODEL/Subsys Handling/Subsystem ==
  u : Inport
  v : Inport  Port=2
  yaw angle : Inport  Port=3
  Add : Sum
  Add1 : Sum  Inputs=+-
  Integrator : Integrator
  Integrator1 : Integrator
  Product{,1..3} (4 alike) : Product  RndMeth=Zero
  Scope : Scope
  Scope1 : Scope
  To Workspace : ToWorkspace  VariableName=Vy_2  SaveFormat=Timeseries  SampleTime=-1
  To Workspace1 : ToWorkspace  VariableName=Vx_2  SaveFormat=Timeseries  SampleTime=-1
  X1 : Scope
  Y1 : Scope
  cos : Trigonometry  Operator=cos
  cos1 : Trigonometry
  X : Outport
  Y : Outport  Port=2
  wires:
  yaw angle/1 -> cos/1, cos1/1
  u/1 -> Product1/1, Product/1
  cos/1 -> Product1/2, Product3/2
  cos1/1 -> Product2/2, Product/2
  v/1 -> Product2/1, Product3/1
  Product1/1 -> Add1/1
  Product2/1 -> Add1/2
  Add1/1 -> Scope/1, To Workspace1/1, Integrator/1  "Vx_2"
  Add/1 -> Scope1/1, To Workspace/1, Integrator1/1  "Vy_2"
  Product3/1 -> Add/2
  Product/1 -> Add/1
  Integrator/1 -> X1/1, X/1
  Integrator1/1 -> Y1/1, Y/1

== system TorqueVectoring_6_1/Vehicle Dynamics Model/14 DOF MODEL/Subsys Tire/Subsys tfl ==
  Slip Ratio : Inport
  Fz : Inport  Port=2
  alpha : Inport  Port=3
  Coeff Rolling Fric : Constant  Value=.02
  Fx Tire : MATLAB Function  TreatAsAtomicUnit=on
  Fy Tire : MATLAB Function  TreatAsAtomicUnit=on
  Gain : Gain
  Gain1 : Gain
  Gain2 : Gain  Gain=180/pi
  Gain3 : Gain  Gain=.001
  Product : Product
  Scope{,1,4,6..7} (5 alike) : Scope
  Subsys Fx : Subsystem  Commented=on
  Subsys Fy : Subsystem  Commented=on
  Subsys Mz : Subsystem
  Subtract1 : Sum  Inputs=+-
  Fx : Outport
  Fy : Outport  Port=2
  Mz : Outport  Port=3
  wires:
  Fz/1 -> Scope6/1, Gain1/1
  alpha/1 -> Gain2/1
  Subsys Fx/1(Fx) -> Scope/1
  Subsys Mz/1(Mz) -> Mz/1
  Gain2/1 -> Fy Tire/1(SA), Scope7/1, Subsys Mz/1(alpha)
  Fx Tire/1(FX) -> Subtract1/1
  Fy Tire/1(FY) -> Fy/1
  Slip Ratio/1 -> Scope1/1, Gain/1
  Subsys Fy/1(Fy) -> ?
  Gain1/1 -> Fx Tire/2(FZ), Product/1, Fy Tire/2(FZ), Gain3/1, Scope4/1
  Gain/1 -> Fx Tire/1(SL)
  Gain3/1 -> Subsys Mz/2(Fz)
  Subtract1/1 -> Fx/1
  Coeff Rolling Fric/1 -> Product/2
  Product/1 -> Subtract1/2

== system TorqueVectoring_6_1/Vehicle Dynamics Model/14 DOF MODEL/Subsys Tire/Subsys tfl1 ==
  S : Inport
  Fz : Inport  Port=2
  alpha : Inport  Port=3
  Coeff Rolling Fric : Constant  Value=.02
  Fx Tire : MATLAB Function  TreatAsAtomicUnit=on
  Fy Tire : MATLAB Function  TreatAsAtomicUnit=on
  Gain1 : Gain  Gain=180/pi
  Gain2 : Gain
  Gain3 : Gain  Gain=.001
  Product : Product
  Scope : Scope
  Subsys Fx : Subsystem  Commented=on
  Subsys Fy : Subsystem  Commented=on
  Subsys Mz : Subsystem
  Subtract1 : Sum  Inputs=+-
  Fx : Outport
  Fy : Outport  Port=2
  Mz : Outport  Port=3
  wires:
  Subsys Fy/1(Fy) -> ?
  Subsys Fx/1(Fx) -> ?
  alpha/1 -> Gain1/1
  Fz/1 -> Gain2/1
  Subsys Mz/1(Mz) -> Mz/1
  Gain1/1 -> Fy Tire/1(SA), Subsys Mz/1(alpha)
  Fx Tire/1(FX) -> Subtract1/1
  Fy Tire/1(FY) -> Fy/1
  S/1 -> Fx Tire/1(SL), Scope/1
  Gain2/1 -> Product/1, Fx Tire/2(FZ), Gain3/1, Fy Tire/2(FZ)
  Gain3/1 -> Subsys Mz/2(Fz)
  Product/1 -> Subtract1/2
  Coeff Rolling Fric/1 -> Product/2
  Subtract1/1 -> Fx/1

== system TorqueVectoring_6_1/Vehicle Dynamics Model/14 DOF MODEL/Subsys Tire/Subsys tfl2 ==
  S : Inport
  Fz : Inport  Port=2
  alpha : Inport  Port=3
  Coeff Rolling Fric : Constant  Value=.02
  Fx Tire : MATLAB Function  TreatAsAtomicUnit=on
  Fy Tire : MATLAB Function  TreatAsAtomicUnit=on
  Gain1 : Gain  Gain=180/pi
  Gain2 : Gain
  Gain3 : Gain  Gain=.001
  Product : Product
  Subsys Fx : Subsystem  Commented=on
  Subsys Fy : Subsystem  Commented=on
  Subsys Mz : Subsystem
  Subtract1 : Sum  Inputs=+-
  Fx : Outport
  Fy : Outport  Port=2
  Mz : Outport  Port=3
  wires:
  Fz/1 -> Gain2/1
  alpha/1 -> Gain1/1
  Subsys Fx/1(Fx) -> ?
  Subsys Fy/1(Fy) -> ?
  Subsys Mz/1(Mz) -> Mz/1
  Gain1/1 -> Fy Tire/1(SA), Subsys Mz/1(alpha)
  Fx Tire/1(FX) -> Subtract1/1
  Fy Tire/1(FY) -> Fy/1
  S/1 -> Fx Tire/1(SL)
  Gain2/1 -> Product/1, Fx Tire/2(FZ), Gain3/1, Fy Tire/2(FZ)
  Gain3/1 -> Subsys Mz/2(Fz)
  Subtract1/1 -> Fx/1
  Product/1 -> Subtract1/2
  Coeff Rolling Fric/1 -> Product/2

== system TorqueVectoring_6_1/Vehicle Dynamics Model/14 DOF MODEL/Subsys Tire/Subsys tfl3 ==
  S : Inport
  Fz : Inport  Port=2
  alpha : Inport  Port=3
  Coeff Rolling Fric : Constant  Value=.02
  Fx Tire : MATLAB Function  TreatAsAtomicUnit=on
  Fy Tire : MATLAB Function  TreatAsAtomicUnit=on
  Gain : Gain
  Gain1 : Gain  Gain=180/pi
  Gain2 : Gain  Gain=.001
  Product : Product
  Subsys Fx : Subsystem  Commented=on
  Subsys Fy : Subsystem  Commented=on
  Subsys Mz : Subsystem
  Subtract1 : Sum  Inputs=+-
  Fx : Outport
  Fy : Outport  Port=2
  Mz : Outport  Port=3
  wires:
  Subsys Mz/1(Mz) -> Mz/1
  Subsys Fy/1(Fy) -> ?
  Subsys Fx/1(Fx) -> ?
  alpha/1 -> Gain1/1
  Fz/1 -> Gain/1
  Gain1/1 -> Fy Tire/1(SA), Subsys Mz/1(alpha)
  Fy Tire/1(FY) -> Fy/1
  S/1 -> Fx Tire/1(SL)
  Fx Tire/1(FX) -> Subtract1/1
  Gain2/1 -> Subsys Mz/2(Fz)
  Product/1 -> Subtract1/2
  Gain/1 -> Product/1, Fx Tire/2(FZ), Gain2/1, Fy Tire/2(FZ)
  Coeff Rolling Fric/1 -> Product/2
  Subtract1/1 -> Fx/1

== system TorqueVectoring_6_1/Vehicle Dynamics Model/14 DOF MODEL/Subsys ride/Ffl ==
  Zufl dot : Inport
  Zsfl dot : Inport  Port=2
  Add : Sum
  Csfl : Gain  Gain=Csfl
  Integrator1 : Integrator
  Integrator2 : Integrator
  Ksfl : Gain  Gain=Ksfl
  Subtract : Sum  Inputs=+-
  Subtract1 : Sum  Inputs=+-
  Ffl : Outport
  wires:
  Zufl dot/1 -> Subtract/1, Integrator1/1
  Subtract/1 -> Csfl/1
  Zsfl dot/1 -> Subtract/2, Integrator2/1
  Subtract1/1 -> Ksfl/1
  Csfl/1 -> Add/1
  Ksfl/1 -> Add/2
  Add/1 -> Ffl/1
  Integrator1/1 -> Subtract1/1
  Integrator2/1 -> Subtract1/2

== system TorqueVectoring_6_1/Vehicle Dynamics Model/14 DOF MODEL/Subsys ride/Ffr ==
  Zufr dot : Inport
  Zsfr dot : Inport  Port=2
  Add : Sum
  Csfr : Gain  Gain=Csfr
  Integrator1 : Integrator
  Integrator2 : Integrator
  Ksfr : Gain  Gain=Ksfr
  Subtract : Sum  Inputs=+-
  Subtract1 : Sum  Inputs=+-
  Ffr : Outport
  wires:
  Add/1 -> Ffr/1
  Ksfr/1 -> Add/2
  Csfr/1 -> Add/1
  Subtract1/1 -> Ksfr/1
  Zsfr dot/1 -> Subtract/2, Integrator2/1
  Subtract/1 -> Csfr/1
  Zufr dot/1 -> Subtract/1, Integrator1/1
  Integrator1/1 -> Subtract1/1
  Integrator2/1 -> Subtract1/2

== system TorqueVectoring_6_1/Vehicle Dynamics Model/14 DOF MODEL/Subsys ride/Frl ==
  Zurl dot : Inport
  Zsrl dot : Inport  Port=2
  Add : Sum
  Csrl : Gain  Gain=Csrl
  Integrator1 : Integrator
  Integrator2 : Integrator
  Ksrl : Gain  Gain=Ksrl
  Subtract : Sum  Inputs=+-
  Subtract1 : Sum  Inputs=+-
  Frl : Outport
  wires:
  Zurl dot/1 -> Subtract/1, Integrator1/1
  Subtract/1 -> Csrl/1
  Zsrl dot/1 -> Subtract/2, Integrator2/1
  Subtract1/1 -> Ksrl/1
  Csrl/1 -> Add/1
  Ksrl/1 -> Add/2
  Add/1 -> Frl/1
  Integrator1/1 -> Subtract1/1
  Integrator2/1 -> Subtract1/2

== system TorqueVectoring_6_1/Vehicle Dynamics Model/14 DOF MODEL/Subsys ride/Frr ==
  Zurr dot : Inport
  Zsrr dot : Inport  Port=2
  Add : Sum
  Csrr : Gain  Gain=Csrr
  Integrator1 : Integrator
  Integrator2 : Integrator
  Ksrr : Gain  Gain=Ksrr
  Subtract : Sum  Inputs=+-
  Subtract1 : Sum  Inputs=+-
  Frr : Outport
  wires:
  Add/1 -> Frr/1
  Ksrr/1 -> Add/2
  Csrr/1 -> Add/1
  Subtract1/1 -> Ksrr/1
  Zsrr dot/1 -> Subtract/2, Integrator2/1
  Subtract/1 -> Csrr/1
  Zurr dot/1 -> Subtract/1, Integrator1/1
  Integrator1/1 -> Subtract1/1
  Integrator2/1 -> Subtract1/2

== system TorqueVectoring_6_1/Vehicle Dynamics Model/14 DOF MODEL/Subsys ride/Subsys Fz ==
  Ffl : Inport
  Ffr : Inport  Port=2
  Frl : Inport  Port=3
  Frr : Inport  Port=4
  Subsys Fzfl : Subsystem
  Subsys Fzfr : Subsystem
  Subsys Fzrl : Subsystem
  Subsys Fzrl1 : Subsystem
  To Workspace : ToWorkspace  VariableName=Fzfl1  SampleTime=-1
  To Workspace1 : ToWorkspace  VariableName=Fzfr1  SampleTime=-1
  To Workspace2 : ToWorkspace  VariableName=Fzrl1  SampleTime=-1
  To Workspace3 : ToWorkspace  VariableName=Fzrr1  SampleTime=-1
  Fzfl : Outport
  Fzfr : Outport  Port=2
  Fzrl : Outport  Port=3
  Fzrr : Outport  Port=4
  wires:
  Ffl/1 -> Subsys Fzfl/1(Ffl)
  Subsys Fzfl/1(Fzfl) -> Fzfl/1, To Workspace/1
  Ffr/1 -> Subsys Fzfr/1(Ffr)
  Subsys Fzfr/1(Fzfr) -> Fzfr/1, To Workspace1/1
  Frl/1 -> Subsys Fzrl/1(Frl)
  Subsys Fzrl/1(Fzrl) -> Fzrl/1, To Workspace2/1
  Frr/1 -> Subsys Fzrl1/1(Frr)
  Subsys Fzrl1/1(Fzrr) -> Fzrr/1, To Workspace3/1

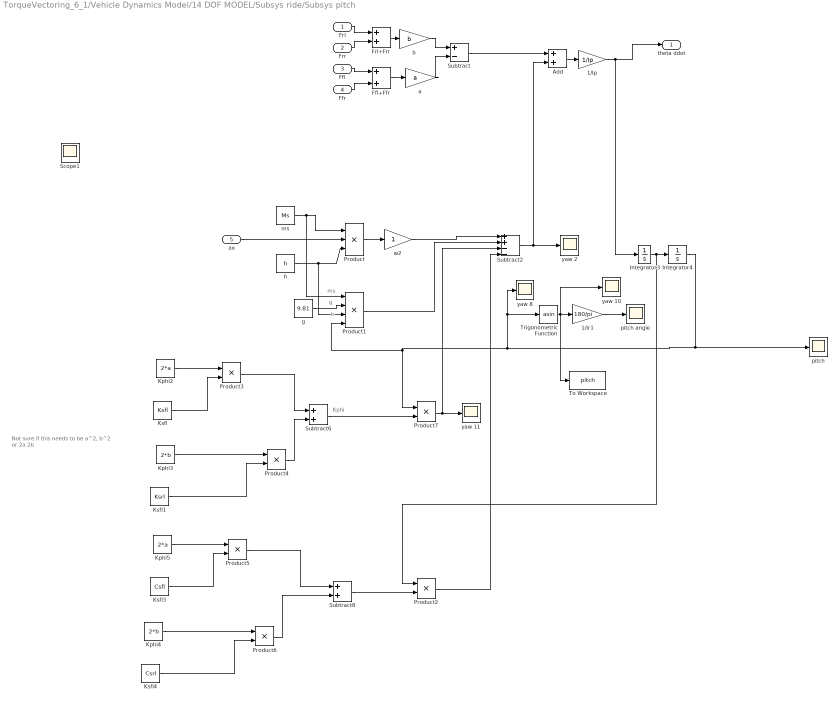
== system TorqueVectoring_6_1/Vehicle Dynamics Model/14 DOF MODEL/Subsys ride/Subsys pitch ==
  note: Kphi
  note: g
  note: ms
  note: h
  note: Not sure if this needs to be a^2, b^2
      | or  2a 2b
  Frl : Inport
  Frr : Inport  Port=2
  Ffl : Inport  Port=3
  Ffr : Inport  Port=4
  ax : Inport  Port=5
  1/Ip : Gain  Gain=1/Ip
  1/Ir1 : Gain  Gain=180/pi
  Add : Sum
  Ffl+Ffr : Sum
  Frl+Frr : Sum
  Integrator3 : Integrator
  Integrator4 : Integrator
  Kphi2 : Constant  Value=2*a
  Kphi3 : Constant  Value=2*b
  Kphi4 : Constant  Value=2*b
  Kphi5 : Constant  Value=2*a
  Ksfl : Constant  Value=Ksfl
  Ksfl1 : Constant  Value=Ksrl
  Ksfl3 : Constant  Value=Csfl
  Ksfl4 : Constant  Value=Csrl
  Product : Product  Inputs=3  RndMeth=Zero
  Product1 : Product  Inputs=4  RndMeth=Zero
  Product{2..7} (6 alike) : Product  RndMeth=Zero
  Scope1 : Scope
  Subtract : Sum  Inputs=+-
  Subtract2 : Sum  Inputs=++--
  Subtract6 : Sum
  Subtract8 : Sum
  To Workspace : ToWorkspace  VariableName=pitch  SampleTime=-1
  Trigonometric Function : Trigonometry  Operator=asin
  a : Gain  Gain=a
  b : Gain  Gain=b
  g : Constant  Value=9.81
  h : Constant  Value=h
  ms : Constant  Value=Ms
  pitch : Scope
  pitch angle : Scope
  w2 : Gain
  yaw {2,8,10..11} (4 alike) : Scope
  theta ddot : Outport
  wires:
  Frl+Frr/1 -> b/1
  Ffl+Ffr/1 -> a/1
  b/1 -> Subtract/1
  a/1 -> Subtract/2
  Frl/1 -> Frl+Frr/1
  Frr/1 -> Frl+Frr/2
  Ffl/1 -> Ffl+Ffr/1
  Ffr/1 -> Ffl+Ffr/2
  ax/1 -> Product/2
  Subtract6/1 -> Product7/2
  h/1 -> Product/3, Product1/3
  Product5/1 -> Subtract8/1
  Product/1 -> w2/1
  Kphi5/1 -> Product5/1
  Product7/1 -> Subtract2/3, yaw 11/1
  Product6/1 -> Subtract8/2
  Ksfl4/1 -> Product6/2
  Kphi2/1 -> Product3/1
  Ksfl1/1 -> Product4/2
  Subtract2/1 -> Add/2, yaw 2/1
  Kphi3/1 -> Product4/1
  w2/1 -> Subtract2/1
  Subtract8/1 -> Product2/2
  Kphi4/1 -> Product6/1
  Ksfl3/1 -> Product5/2
  Product3/1 -> Subtract6/1
  g/1 -> Product1/2
  1/Ir1/1 -> pitch angle/1
  Trigonometric Function/1 -> 1/Ir1/1, yaw 10/1, To Workspace/1
  Ksfl/1 -> Product3/2
  Product1/1 -> Subtract2/2
  Product4/1 -> Subtract6/2
  ms/1 -> Product/1, Product1/1
  Product2/1 -> Subtract2/4
  Subtract/1 -> Add/1
  Add/1 -> 1/Ip/1
  1/Ip/1 -> Integrator3/1, theta ddot/1
  Integrator4/1 -> Product1/4, Product7/1, Trigonometric Function/1, yaw 8/1, pitch/1
  Integrator3/1 -> Product2/1, Integrator4/1

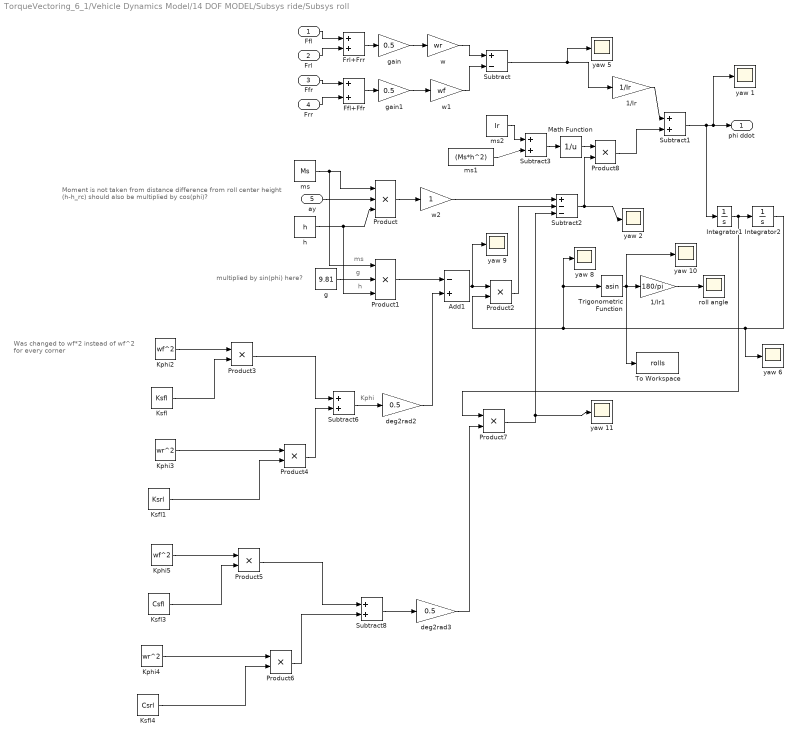
== system TorqueVectoring_6_1/Vehicle Dynamics Model/14 DOF MODEL/Subsys ride/Subsys roll ==
  note: Moment is not taken from distance difference from roll center height
      | (h-h_rc)
      | should also be multiplied by cos(phi)?
  note: g
  note: ms
  note: h
  note: Kphi
  note: Was changed to wf*2 instead of wf^2
      | for every corner
  note: multiplied by sin(phi) here?
  Ffl : Inport
  Frl : Inport  Port=2
  Ffr : Inport  Port=3
  Frr : Inport  Port=4
  ay : Inport  Port=5
  1/Ir : Gain  Gain=1/Ir
  1/Ir1 : Gain  Gain=180/pi
  Add1 : Sum  Inputs=-+
  Ffl+Ffr : Sum
  Frl+Frr : Sum
  Integrator1 : Integrator
  Integrator2 : Integrator
  Kphi2 : Constant  Value=wf^2
  Kphi3 : Constant  Value=wr^2
  Kphi4 : Constant  Value=wr^2
  Kphi5 : Constant  Value=wf^2
  Ksfl : Constant  Value=Ksfl
  Ksfl1 : Constant  Value=Ksrl
  Ksfl3 : Constant  Value=Csfl
  Ksfl4 : Constant  Value=Csrl
  Math Function : Math  Operator=reciprocal  SignedPower=on
  Product : Product  Inputs=3  RndMeth=Zero
  Product1 : Product  Inputs=3  RndMeth=Zero
  Product{2..8} (7 alike) : Product  RndMeth=Zero
  Subtract : Sum  Inputs=+-
  Subtract{1,3,6,8} (4 alike) : Sum
  Subtract2 : Sum  Inputs=+--
  To Workspace : ToWorkspace  VariableName=rolls  SampleTime=-1
  Trigonometric Function : Trigonometry  Operator=asin
  deg2rad2 : Gain  Gain=0.5
  deg2rad3 : Gain  Gain=0.5
  g : Constant  Value=9.81
  gain : Gain  Gain=0.5
  gain1 : Gain  Gain=0.5
  h : Constant  Value=h
  ms : Constant  Value=Ms
  ms1 : Constant  Value=(Ms*h^2)
  ms2 : Constant  Value=Ir
  roll angle : Scope
  w : Gain  Gain=wr
  w1 : Gain  Gain=wf
  w2 : Gain
  yaw {1..2,5..6,8..11} (8 alike) : Scope
  phi ddot : Outport
  wires:
  Frr/1 -> Ffl+Ffr/2
  Ffr/1 -> Ffl+Ffr/1
  Frl/1 -> Frl+Frr/2
  Ffl/1 -> Frl+Frr/1
  Subtract/1 -> yaw 5/1, 1/Ir/1
  Ffl+Ffr/1 -> gain1/1
  Frl+Frr/1 -> gain/1
  gain/1 -> w/1
  gain1/1 -> w1/1
  w/1 -> Subtract/1
  w1/1 -> Subtract/2
  ms/1 -> Product/1, Product1/1
  h/1 -> Product/3, Product1/3
  g/1 -> Product1/2
  Add1/1 -> Product2/1, yaw 9/1
  Product/1 -> w2/1
  ay/1 -> Product/2
  Subtract2/1 -> yaw 2/1, Product8/2
  Integrator1/1 -> Integrator2/1, Product7/1
  Product2/1 -> Subtract2/2
  Integrator2/1 -> Product2/2, Trigonometric Function/1, yaw 8/1, yaw 6/1
  Subtract1/1 -> phi ddot/1, yaw 1/1, Integrator1/1
  Trigonometric Function/1 -> 1/Ir1/1, yaw 10/1, To Workspace/1
  1/Ir1/1 -> roll angle/1
  Ksfl/1 -> Product3/2
  Kphi2/1 -> Product3/1
  Ksfl1/1 -> Product4/2
  Kphi3/1 -> Product4/1
  Ksfl3/1 -> Product5/2
  Kphi5/1 -> Product5/1
  Product3/1 -> Subtract6/1
  Product4/1 -> Subtract6/2
  Ksfl4/1 -> Product6/2
  Kphi4/1 -> Product6/1
  Product6/1 -> Subtract8/2
  Product5/1 -> Subtract8/1
  Subtract8/1 -> deg2rad3/1
  Product7/1 -> yaw 11/1, Subtract2/3
  Subtract6/1 -> deg2rad2/1
  ms2/1 -> Subtract3/1
  ms1/1 -> Subtract3/2
  1/Ir/1 -> Subtract1/1
  Subtract3/1 -> Math Function/1
  Product8/1 -> Subtract1/2
  Math Function/1 -> Product8/1
  deg2rad2/1 -> Add1/2
  deg2rad3/1 -> Product7/2
  w2/1 -> Subtract2/1
  Product1/1 -> Add1/1

== system TorqueVectoring_6_1/Vehicle Dynamics Model/14 DOF MODEL/Subsys ride/Subsys sprung vertical ==
  Ffl : Inport
  Ffr : Inport  Port=2
  Frl : Inport  Port=3
  Frr : Inport  Port=4
  ay : Inport  Port=5
  Add : Sum  Inputs=+++++
  Gain : Gain  Gain=1/Ms
  Gain1 : Gain  Gain=Ms*h*2/wf
  Math Function1 : Math  Operator=square  SignedPower=on
  Zs ddot : Outport
  wires:
  Add/1 -> Gain/1
  Ffl/1 -> Add/1
  Ffr/1 -> Add/2
  Gain/1 -> Zs ddot/1
  Frl/1 -> Add/3
  Frr/1 -> Add/4
  ay/1 -> Gain1/1
  Gain1/1 -> Add/5

== system TorqueVectoring_6_1/Vehicle Dynamics Model/14 DOF MODEL/Subsys ride/Subsys wheel fl ==
  Zufl : Inport
  Ffl : Inport  Port=2
  Zrfl : Inport  Port=3
  Divide : Product  Inputs=*/
  Ftfl : Subsystem
  Subtract : Sum  Inputs=+-
  mufl : Constant  Value=mufl
  Zufl ddot : Outport
  wires:
  Zrfl/1 -> Ftfl/1(Zrfl)
  Ftfl/1(Ftfl) -> Subtract/1
  Zufl/1 -> Ftfl/2(Zufl)
  Ffl/1 -> Subtract/2
  Subtract/1 -> Divide/1
  mufl/1 -> Divide/2
  Divide/1 -> Zufl ddot/1

== system TorqueVectoring_6_1/Vehicle Dynamics Model/14 DOF MODEL/Subsys ride/Subsys wheel fr ==
  Zufr : Inport
  Ffr : Inport  Port=2
  Zrfr : Inport  Port=3
  Divide : Product  Inputs=*/
  Ftfr : Subsystem
  Subtract1 : Sum  Inputs=+-
  mufr : Constant  Value=mufr
  Zufr ddot : Outport
  wires:
  Zrfr/1 -> Ftfr/1(Zrfr)
  Ftfr/1(Ftfr) -> Subtract1/1
  Zufr/1 -> Ftfr/2(Zufr)
  Ffr/1 -> Subtract1/2
  Subtract1/1 -> Divide/1
  mufr/1 -> Divide/2
  Divide/1 -> Zufr ddot/1

== system TorqueVectoring_6_1/Vehicle Dynamics Model/14 DOF MODEL/Subsys ride/Subsys wheel rl ==
  Zurl : Inport
  Frl : Inport  Port=2
  Zrrl : Inport  Port=3
  Divide : Product  Inputs=*/
  Ftrl : Subsystem
  Subtract2 : Sum  Inputs=+-
  murl : Constant  Value=murl
  Zurl ddot : Outport
  wires:
  Zrrl/1 -> Ftrl/1(Zrrl)
  Ftrl/1(Ftrl) -> Subtract2/1
  Zurl/1 -> Ftrl/2(Zurl)
  Frl/1 -> Subtract2/2
  Subtract2/1 -> Divide/1
  murl/1 -> Divide/2
  Divide/1 -> Zurl ddot/1

== system TorqueVectoring_6_1/Vehicle Dynamics Model/14 DOF MODEL/Subsys ride/Subsys wheel rr ==
  Zurr : Inport
  Frr : Inport  Port=2
  Zrrr : Inport  Port=3
  Divide : Product  Inputs=*/
  Ftfr2 : Subsystem
  Subtract3 : Sum  Inputs=+-
  murr : Constant  Value=murr
  Zurr ddot : Outport
  wires:
  Zrrr/1 -> Ftfr2/1(Zrrr)
  Ftfr2/1(Ftfr) -> Subtract3/1
  Zurr/1 -> Ftfr2/2(Zurr)
  Frr/1 -> Subtract3/2
  Subtract3/1 -> Divide/1
  murr/1 -> Divide/2
  Divide/1 -> Zurr ddot/1

== system TorqueVectoring_6_1/Vehicle Dynamics Model/14 DOF MODEL/Subsys ride/Zsfl dot ==
  Zs dot : Inport
  thita dot : Inport  Port=2
  chi dot : Inport  Port=3
  0.5 : Gain  Gain=0.5
  Add : Sum  Inputs=+-+
  a : Gain  Gain=a
  wfl : Gain  Gain=wf
  Zsfl dot : Outport
  wires:
  Zs dot/1 -> Add/1
  a/1 -> Add/2
  thita dot/1 -> a/1
  wfl/1 -> Add/3
  chi dot/1 -> 0.5/1
  Add/1 -> Zsfl dot/1
  0.5/1 -> wfl/1

== system TorqueVectoring_6_1/Vehicle Dynamics Model/14 DOF MODEL/Subsys ride/Zsfr dot ==
  Zs dot : Inport
  thita dot : Inport  Port=2
  chi dot : Inport  Port=3
  0.5 : Gain  Gain=0.5
  Add : Sum  Inputs=+--
  a : Gain  Gain=a
  w : Gain  Gain=wf
  Zsfr dot : Outport
  wires:
  Add/1 -> Zsfr dot/1
  chi dot/1 -> 0.5/1
  w/1 -> Add/3
  thita dot/1 -> a/1
  a/1 -> Add/2
  Zs dot/1 -> Add/1
  0.5/1 -> w/1

== system TorqueVectoring_6_1/Vehicle Dynamics Model/14 DOF MODEL/Subsys ride/Zsrl dot ==
  Zs dot : Inport
  thita dot : Inport  Port=2
  chi dot : Inport  Port=3
  0.5 : Gain  Gain=0.5
  Add : Sum  Inputs=+++
  b : Gain  Gain=b
  w : Gain  Gain=wr
  Zsrl dot : Outport
  wires:
  Zs dot/1 -> Add/1
  b/1 -> Add/2
  thita dot/1 -> b/1
  w/1 -> Add/3
  0.5/1 -> w/1
  chi dot/1 -> 0.5/1
  Add/1 -> Zsrl dot/1

== system TorqueVectoring_6_1/Vehicle Dynamics Model/14 DOF MODEL/Subsys ride/Zsrr dot ==
  Zs dot : Inport
  thita dot : Inport  Port=2
  chi dot : Inport  Port=3
  0.5 : Gain  Gain=0.5
  Add : Sum  Inputs=++-
  b : Gain  Gain=b
  w : Gain  Gain=wr
  Zsrr dot : Outport
  wires:
  Add/1 -> Zsrr dot/1
  chi dot/1 -> 0.5/1
  0.5/1 -> w/1
  w/1 -> Add/3
  thita dot/1 -> b/1
  b/1 -> Add/2
  Zs dot/1 -> Add/1

== system TorqueVectoring_6_1/Vehicle Dynamics Model/14 DOF MODEL/Subsys Tire/Subsys tfl/Subsys Fx ==
  note: note
      | Coefficient values generated from Arash Tire Parser
  note: B
  note: Bx
  note: Bx - atanBX
  note: X
  note: x
  S : Inport
  Fz : Inport  Port=2
  Bx : Product  RndMeth=Zero
  C : Constant  Value=9.024117283527670e-04
  Divide : Product  Inputs=*/
  Gain : Gain  Gain=100
  Product{1..4} (4 alike) : Product  RndMeth=Zero
  Scope2 : Scope
  Sh2 : Constant  Value=0
  Subsys BCD (Cornering Stiffness) : Subsystem
  Subsys D : Subsystem
  SubsysE : Subsystem
  Subtract : Sum  Inputs=+-
  Subtract1 : Sum  Inputs=+-
  Subtract3 : Sum
  Subtract4 : Sum
  Sv : Constant  Value=0
  To Workspace1 : ToWorkspace  VariableName=Fxfls  SampleTime=-1
  atan : Trigonometry  Operator=atan
  atanBx : Trigonometry  Operator=atan
  atanBx1 : Trigonometry
  Fx : Outport
  wires:
  C/1 -> Product2/1, Product3/2
  Subsys D/1(D) -> Product2/2, Product4/2
  Subsys BCD (Cornering Stiffness)/1(BCD) -> Divide/1
  Product2/1 -> Divide/2
  Subtract3/1 -> Scope2/1, To Workspace1/1, Fx/1
  Product4/1 -> Subtract3/1
  Product3/1 -> atanBx1/1
  atanBx1/1 -> Product4/1
  atan/1 -> Product3/1
  S/1 -> Gain/1
  Subtract4/1 -> Bx/1
  Sv/1 -> Subtract3/2
  Subtract1/1 -> atan/1
  Product1/1 -> Subtract1/2
  SubsysE/1(E) -> Product1/2
  Subtract/1 -> Product1/1
  atanBx/1 -> Subtract/2
  Bx/1 -> Subtract/1, Subtract1/1, atanBx/1
  Divide/1 -> Bx/2
  Sh2/1 -> Subtract4/2
  Fz/1 -> Subsys BCD (Cornering Stiffness)/1(Fz), Subsys D/1(Fz)
  Gain/1 -> Subtract4/1

== system TorqueVectoring_6_1/Vehicle Dynamics Model/14 DOF MODEL/Subsys Tire/Subsys tfl/Subsys Fy ==
  note: B
  note: Bx
  note: Bx - atanBX
  note: X
  note: x
  note: Sh
  alpha : Inport
  Fz : Inport  Port=2
  Bx : Product  RndMeth=Zero
  C : Constant  Value=1.3
  Divide : Product  Inputs=*/
  Product{1..4} (4 alike) : Product  RndMeth=Zero
  Scope2 : Scope
  Subsys BCD : Subsystem
  Subsys D : Subsystem
  SubsysE : Subsystem
  Subtract : Sum  Inputs=+-
  Subtract1 : Sum  Inputs=+-
  Subtract3 : Sum
  Subtract4 : Sum
  Sv : Constant  Value=0
  Sv1 : Constant  Value=0
  To Workspace1 : ToWorkspace  VariableName=Fyfls  SampleTime=-1
  atan : Trigonometry  Operator=atan
  atanBx : Trigonometry  Operator=atan
  atanBx1 : Trigonometry
  Fy : Outport
  wires:
  C/1 -> Product2/1, Product3/2
  Subsys D/1(D) -> Product2/2, Product4/2
  Product2/1 -> Divide/2
  Subtract3/1 -> To Workspace1/1, Fy/1, Scope2/1
  Product4/1 -> Subtract3/1
  Product3/1 -> atanBx1/1
  atanBx1/1 -> Product4/1
  atan/1 -> Product3/1
  Subtract4/1 -> Bx/1
  Sv/1 -> Subtract3/2
  Subtract1/1 -> atan/1
  Product1/1 -> Subtract1/2
  SubsysE/1(E) -> Product1/2
  Subtract/1 -> Product1/1
  atanBx/1 -> Subtract/2
  Bx/1 -> Subtract/1, Subtract1/1, atanBx/1
  Divide/1 -> Bx/2
  Sv1/1 -> Subtract4/2
  Subsys BCD/1(BCD) -> Divide/1
  alpha/1 -> Subtract4/1
  Fz/1 -> Subsys BCD/1(Fz), Subsys D/1(Fz), SubsysE/1(Fz)

== system TorqueVectoring_6_1/Vehicle Dynamics Model/14 DOF MODEL/Subsys Tire/Subsys tfl/Subsys Mz ==
  note: B
  note: Bx
  note: Bx - atanBX
  note: X
  note: x
  alpha : Inport
  Fz : Inport  Port=2
  Bx : Product  RndMeth=Zero
  C : Constant  Value=2.40
  Divide : Product  Inputs=*/
  Product{1..4} (4 alike) : Product  RndMeth=Zero
  Scope2 : Scope
  Sh2 : Constant  Value=0
  Subsys BCD : Subsystem
  Subsys D : Subsystem
  SubsysE : Subsystem
  Subtract : Sum  Inputs=+-
  Subtract1 : Sum  Inputs=+-
  Subtract3 : Sum
  Subtract4 : Sum
  Sv2 : Constant  Value=0
  To Workspace1 : ToWorkspace  VariableName=Mzfls  SampleTime=-1
  atan : Trigonometry  Operator=atan
  atanBx : Trigonometry  Operator=atan
  atanBx1 : Trigonometry
  Mz : Outport
  wires:
  C/1 -> Product2/1, Product3/2
  Subsys D/1(D) -> Product2/2, Product4/2
  Subsys BCD/1(BCD) -> Divide/1
  Product2/1 -> Divide/2
  Subtract3/1 -> Scope2/1, To Workspace1/1, Mz/1
  Product4/1 -> Subtract3/1
  Product3/1 -> atanBx1/1
  atanBx1/1 -> Product4/1
  atan/1 -> Product3/1
  alpha/1 -> Subtract4/1
  Subtract4/1 -> Bx/1
  Sv2/1 -> Subtract3/2
  Subtract1/1 -> atan/1
  Product1/1 -> Subtract1/2
  SubsysE/1(E) -> Product1/2
  Subtract/1 -> Product1/1
  atanBx/1 -> Subtract/2
  Bx/1 -> Subtract/1, Subtract1/1, atanBx/1
  Divide/1 -> Bx/2
  Sh2/1 -> Subtract4/2
  Fz/1 -> Subsys BCD/1(Fz), Subsys D/1(Fz), SubsysE/1(Fz)

== system TorqueVectoring_6_1/Vehicle Dynamics Model/14 DOF MODEL/Subsys Tire/Subsys tfl1/Subsys Fx ==
  note: x
  note: X
  note: Bx - atanBX
  note: Bx
  note: B
  S : Inport
  Fz : Inport  Port=2
  Bx : Product  RndMeth=Zero
  C : Constant  Value=1.65
  Divide : Product  Inputs=*/
  Gain : Gain  Gain=100
  Product{1..4} (4 alike) : Product  RndMeth=Zero
  Scope2 : Scope
  Sh2 : Constant  Value=0
  Subsys BCD : Subsystem
  Subsys D : Subsystem
  SubsysE : Subsystem
  Subtract : Sum  Inputs=+-
  Subtract1 : Sum  Inputs=+-
  Subtract3 : Sum
  Subtract4 : Sum
  Sv : Constant  Value=0
  To Workspace1 : ToWorkspace  VariableName=Fxfrs  SampleTime=-1
  atan : Trigonometry  Operator=atan
  atanBx : Trigonometry  Operator=atan
  atanBx1 : Trigonometry
  Fx : Outport
  wires:
  Gain/1 -> Subtract4/1
  Fz/1 -> SubsysE/1(Fz), Subsys D/1(Fz), Subsys BCD/1(Fz)
  Sh2/1 -> Subtract4/2
  Divide/1 -> Bx/2
  Bx/1 -> atanBx/1, Subtract1/1, Subtract/1
  atanBx/1 -> Subtract/2
  Subtract/1 -> Product1/1
  SubsysE/1(E) -> Product1/2
  Product1/1 -> Subtract1/2
  Subtract1/1 -> atan/1
  Sv/1 -> Subtract3/2
  Subtract4/1 -> Bx/1
  S/1 -> Gain/1
  atan/1 -> Product3/1
  atanBx1/1 -> Product4/1
  Product3/1 -> atanBx1/1
  Product4/1 -> Subtract3/1
  Subtract3/1 -> To Workspace1/1, Fx/1, Scope2/1
  Product2/1 -> Divide/2
  Subsys BCD/1(BCD) -> Divide/1
  Subsys D/1(D) -> Product4/2, Product2/2
  C/1 -> Product3/2, Product2/1

== system TorqueVectoring_6_1/Vehicle Dynamics Model/14 DOF MODEL/Subsys Tire/Subsys tfl1/Subsys Fy ==
  note: Sh
  note: x
  note: X
  note: Bx - atanBX
  note: Bx
  note: B
  alpha : Inport
  Fz : Inport  Port=2
  Bx : Product  RndMeth=Zero
  C : Constant  Value=1.3
  Divide : Product  Inputs=*/
  Product{1..4} (4 alike) : Product  RndMeth=Zero
  Scope2 : Scope
  Subsys BCD : Subsystem
  Subsys D : Subsystem
  SubsysE : Subsystem
  Subtract : Sum  Inputs=+-
  Subtract1 : Sum  Inputs=+-
  Subtract3 : Sum
  Subtract4 : Sum
  Sv : Constant  Value=0
  Sv1 : Constant  Value=0
  To Workspace1 : ToWorkspace  VariableName=Fyfrs  SampleTime=-1
  atan : Trigonometry  Operator=atan
  atanBx : Trigonometry  Operator=atan
  atanBx1 : Trigonometry
  Fy : Outport
  wires:
  Fz/1 -> SubsysE/1(Fz), Subsys D/1(Fz), Subsys BCD/1(Fz)
  alpha/1 -> Subtract4/1
  Subsys BCD/1(BCD) -> Divide/1
  Sv1/1 -> Subtract4/2
  Divide/1 -> Bx/2
  Bx/1 -> atanBx/1, Subtract1/1, Subtract/1
  atanBx/1 -> Subtract/2
  Subtract/1 -> Product1/1
  SubsysE/1(E) -> Product1/2
  Product1/1 -> Subtract1/2
  Subtract1/1 -> atan/1
  Sv/1 -> Subtract3/2
  Subtract4/1 -> Bx/1
  atan/1 -> Product3/1
  atanBx1/1 -> Product4/1
  Product3/1 -> atanBx1/1
  Product4/1 -> Subtract3/1
  Subtract3/1 -> Fy/1, To Workspace1/1, Scope2/1
  Product2/1 -> Divide/2
  Subsys D/1(D) -> Product4/2, Product2/2
  C/1 -> Product3/2, Product2/1

== system TorqueVectoring_6_1/Vehicle Dynamics Model/14 DOF MODEL/Subsys Tire/Subsys tfl1/Subsys Mz ==
  note: x
  note: X
  note: Bx - atanBX
  note: Bx
  note: B
  alpha : Inport
  Fz : Inport  Port=2
  Bx : Product  RndMeth=Zero
  C : Constant  Value=2.40
  Divide : Product  Inputs=*/
  Product{1..4} (4 alike) : Product  RndMeth=Zero
  Scope2 : Scope
  Sh2 : Constant  Value=0
  Subsys BCD : Subsystem
  Subsys D : Subsystem
  SubsysE : Subsystem
  Subtract : Sum  Inputs=+-
  Subtract1 : Sum  Inputs=+-
  Subtract3 : Sum
  Subtract4 : Sum
  Sv2 : Constant  Value=0
  To Workspace1 : ToWorkspace  VariableName=Mzfrs  SampleTime=-1
  atan : Trigonometry  Operator=atan
  atanBx : Trigonometry  Operator=atan
  atanBx1 : Trigonometry
  Mz : Outport
  wires:
  Fz/1 -> SubsysE/1(Fz), Subsys D/1(Fz), Subsys BCD/1(Fz)
  Sh2/1 -> Subtract4/2
  Divide/1 -> Bx/2
  Bx/1 -> atanBx/1, Subtract1/1, Subtract/1
  atanBx/1 -> Subtract/2
  Subtract/1 -> Product1/1
  SubsysE/1(E) -> Product1/2
  Product1/1 -> Subtract1/2
  Subtract1/1 -> atan/1
  Sv2/1 -> Subtract3/2
  Subtract4/1 -> Bx/1
  alpha/1 -> Subtract4/1
  atan/1 -> Product3/1
  atanBx1/1 -> Product4/1
  Product3/1 -> atanBx1/1
  Product4/1 -> Subtract3/1
  Subtract3/1 -> Mz/1, To Workspace1/1, Scope2/1
  Product2/1 -> Divide/2
  Subsys BCD/1(BCD) -> Divide/1
  Subsys D/1(D) -> Product4/2, Product2/2
  C/1 -> Product3/2, Product2/1
